simulink model "tire_model"  (R2024a)
settings: Solver=VariableStepAuto  StartTime=0.0  StopTime=10  RelTol=1e-3
values from neighbouring files (symbols this model uses):
  B = 10    [new-sim-workspace.mat]    (also in workspace-var-complete-jan.mat; workspace-vars.mat; workspace_var_dec_2024.mat; workspace_var_jan_2024.mat)
  C = 1.9    [new-sim-workspace.mat]    (also in workspace-var-complete-jan.mat; workspace-vars.mat; workspace_var_dec_2024.mat; workspace_var_jan_2024.mat)
  D = 1    [new-sim-workspace.mat]    (also in workspace-var-complete-jan.mat; workspace-vars.mat; workspace_var_dec_2024.mat; workspace_var_jan_2024.mat)
  g = 9.81    [new-sim-workspace.mat]    (also in workspace-var-complete-jan.mat; workspace-vars.mat; workspace_var_dec_2024.mat; workspace_var_jan_2024.mat)
  J_w = 0.5    [new-sim-workspace.mat]    (also in workspace-var-complete-jan.mat; workspace-vars.mat; workspace_var_dec_2024.mat; workspace_var_jan_2024.mat)
  M = 100    [new-sim-workspace.mat]    (also in workspace-var-complete-jan.mat; workspace-vars.mat; workspace_var_dec_2024.mat; workspace_var_jan_2024.mat)
  R = 0.5    [new-sim-workspace.mat]    (also in workspace-var-complete-jan.mat; workspace-vars.mat; workspace_var_dec_2024.mat; workspace_var_jan_2024.mat)
settings Model: Creator=kyle  LastModifiedBy=kyle

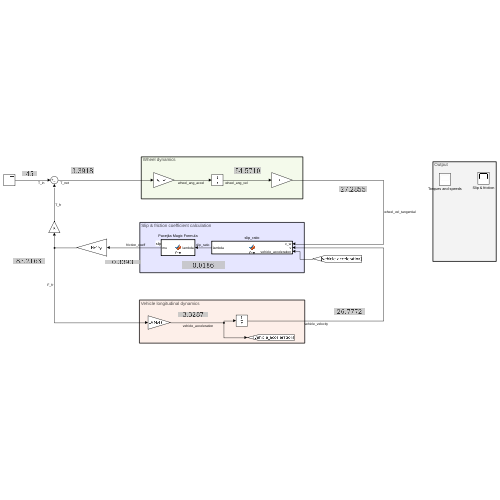
[thumbnail: Simulink's stored preview of the top-level diagram]
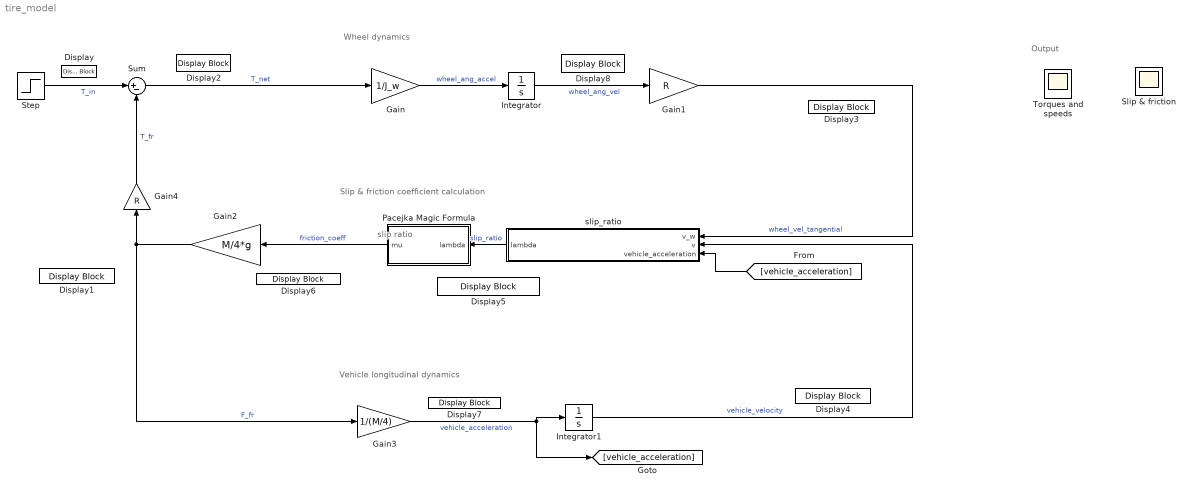
== system tire_model ==
  note: slip ratio
  note: Slip & friction coefficient calculation
  note: Wheel dynamics
  note: Vehicle longitudinal dynamics
  note: Output
  Display{,1..8} (9 alike) : DisplayBlock  LabelPosition=Hide  Transparency=1
  Gain : Gain  Gain=1/J_w
  Gain1 : Gain  Gain=R
  Gain2 : Gain  Gain=M/4*g
  Gain3 : Gain  Gain=1/(M/4)
  Gain4 : Gain  Gain=R
  Integrator : Integrator
  Integrator1 : Integrator
  Pacejka Magic Formula : MATLAB Function  TreatAsAtomicUnit=on
  Slip & friction : Scope
      settings: Floating=on
  Step : Step  Time=2  Before=1  After=45  SampleTime=0
  Sum : Sum  Inputs=|+-
  Torques and speeds : Scope
      settings: Floating=on
  slip_ratio : MATLAB Function  TreatAsAtomicUnit=on
  wires:
  Gain4/1 -> Sum/2  "T_fr"
  [vehicle_acceleration] -> slip_ratio/3(vehicle_acceleration)
  Gain2/1 -> Gain3/1, Gain4/1  "F_fr"
  Integrator/1 -> Gain1/1  "wheel_ang_vel"
  Gain/1 -> Integrator/1  "wheel_ang_accel"
  Pacejka Magic Formula/1(mu) -> Gain2/1  "friction_coeff"
  Sum/1 -> Gain/1  "T_net"
  Step/1 -> Sum/1  "T_in"
  slip_ratio/1(lambda) -> Pacejka Magic Formula/1(lambda)  "slip_ratio"
  Gain1/1 -> slip_ratio/1(v_w)  "wheel_vel_tangential"
  Gain3/1 -> Integrator1/1, [vehicle_acceleration]  "vehicle_acceleration"
  Integrator1/1 -> slip_ratio/2(v)  "vehicle_velocity"

== matlab function tire_model/Pacejka Magic Formula ==
  data: lambda input double size=1; mu output double size=1; B parameter double size=1; C parameter double size=1; D parameter double size=1; E parameter double size=1
function mu = fcn(lambda,B, C, D, E)

mu = D*sin(C*atan(B*lambda -  E*(B*lambda - atan(B*lambda))));

== matlab function tire_model/slip_ratio ==
  data: v_w input; lambda output; v input; TOL parameter; vehicle_acceleration input
function lambda = fcn(v_w, v, TOL, vehicle_acceleration)
% This is derived from pg. 100 of Rajamani - Vehicle Dynamics and Control
% (2006)
eps = 0.00001
if vehicle_acceleration >= 0
    lambda = (v_w - v)/(v_w + eps);
else
    lambda = (v_w - v)/(v + eps);
end
